simulink model "resposta_degrau_pendulo"  (Simulink 7.4)
settings: Solver=ode45  StartTime=0.0  StopTime=5  RelTol=1e-3
StopFcn:
  | disp('O primeiro ponto de g nao eh armazenado !')
  | g = g(2:end);
  | figure,stem(g),title('g(n)'),xlabel('n')
undefined symbols (not defined in the file or in its folder): b, grav, L, m, T, yp_equilibrio
settings Model: Creator=Kawakami  LastModifiedBy=Kawakami
settings DataIOCC: SignalLoggingName=sigsOut
settings DebuggingCC: SaveWithParameterizedLinksMsg=none  SignalResolutionControl=TryResolveAllWithWarning  SolverPrmCheckMsg=none  MultiTaskDSMMsg=warning  MultiTaskCondExecSysMsg=none  StrictBusMsg=None
settings HardwareCC: TargetUnknown=on
settings RTWCC: IncludeERTFirstTime=on

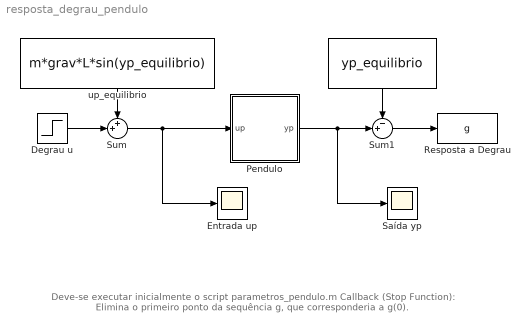
== system resposta_degrau_pendulo ==
  note: Deve-se executar inicialmente o script parametros_pendulo.m
      |
      | Callback (Stop Function):
      | Elimina o primeiro ponto da sequência g, que corresponderia a g(0).
  " " : Constant  Value=yp_equilibrio  OutDataType=sfix(16)  OutScaling=2^0
  Degrau u : Step  Time=0  SampleTime=0
  Entrada up : Scope
  Pendulo : Subsystem  mask{m=m, L=L, grav=grav, b=b, theta0=yp_equilibrio}
      mask prompts: m "m (kg)"; L "L (m)"; grav "grav (m/s^2)"; b "b (Ns/(m*rad))"; theta0 "theta inicial (rad)"
  Resposta a Degrau : ToWorkspace  VariableName=g  SampleTime=T  SaveFormat=Array
  Saída yp : Scope
      settings: TimeRange=5  YMin=0.75  YMax=1
  Sum : Sum  Inputs=++|  OutDataType=sfix(16)  OutScaling=2^0  SaturateOnIntegerOverflow=on
  Sum1 : Sum  Inputs=-+|  OutDataType=sfix(16)  OutScaling=2^0  SaturateOnIntegerOverflow=on
  up_equilibrio : Constant  Value=m*grav*L*sin(yp_equilibrio)  OutDataType=sfix(16)  OutScaling=2^0
  wires:
  Degrau u/1 -> Sum/2
  up_equilibrio/1 -> Sum/1
  Sum/1 -> Pendulo/1(up), Entrada up/1
  " "/1 -> Sum1/1
  Pendulo/1(yp) -> Sum1/2, Saída yp/1
  Sum1/1 -> Resposta a Degrau/1

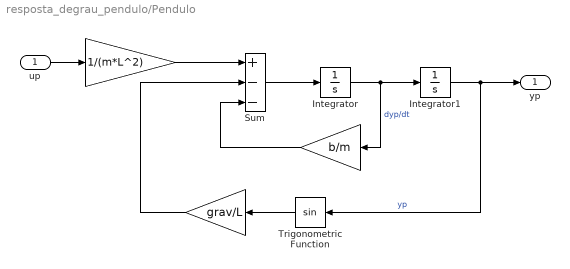
== system resposta_degrau_pendulo/Pendulo ==
  up : Inport  OutDataType=sfix(16)  OutScaling=2^0
  " " : Gain  Gain=b/m  ParameterDataType=sfix(16)  ParameterScaling=2^0  OutDataType=sfix(16)  OutScaling=2^0  SaturateOnIntegerOverflow=on  OutDataTypeStr=Inherit: Same as input  ParamDataTypeStr=Inherit: Same as input
  "  " : Gain  Gain=grav/L  ParameterDataType=sfix(16)  ParameterScaling=2^0  OutDataType=sfix(16)  OutScaling=2^0  SaturateOnIntegerOverflow=on  OutDataTypeStr=Inherit: Same as input  ParamDataTypeStr=Inherit: Same as input
  "   " : Gain  Gain=1/(m*L^2)  ParameterDataType=sfix(16)  ParameterScaling=2^0  OutDataType=sfix(16)  OutScaling=2^0  SaturateOnIntegerOverflow=on  OutDataTypeStr=Inherit: Same as input  ParamDataTypeStr=Inherit: Same as input
  Integrator : Integrator
  Integrator1 : Integrator  InitialCondition=theta0
  Sum : Sum  Inputs=+--  OutDataType=sfix(16)  OutScaling=2^0  SaturateOnIntegerOverflow=on
  Trigonometric Function : Trigonometry
  yp : Outport
  wires:
  Integrator/1 -> Integrator1/1, " "/1  "dyp/dt"
  Sum/1 -> Integrator/1
  "   "/1 -> Sum/1
  Trigonometric Function/1 -> "  "/1
  Integrator1/1 -> Trigonometric Function/1, yp/1  "yp"
  "  "/1 -> Sum/2
  " "/1 -> Sum/3
  up/1 -> "   "/1
